simulink model "ve_model2"  (R2019a)
settings: Solver=FixedStepAuto  StartTime=0.0  StopTime=SimulationTime  FixedStep=IntegrationStep  RelTol=1e-3
model workspace (MAT data in the model file):
  IntegrationStep = 0.1
  SimulationTime = 0.1
  X0 = 0
  X_0 = 0
  Y0 = 0
  Y_0 = 0
  ang = 0.19739555985
  m = 1000
  vel = 3.14159265359
  xinitial = 1
libraries: autolibshared x1
settings Model: Creator=Vikas  LastModifiedBy=Vikas
settings DataIOCC: InitialState=xoutnew  LoadInitialState=on  SaveFinalState=on  SaveOperatingPoint=on  SaveState=on  StateSaveName=xoutnew  OutputSaveName=youtNew  ReturnWorkspaceOutputsName=SDOSimTest_Log
settings DebuggingCC: ArithmeticOperatorsInVariantConditions=warning

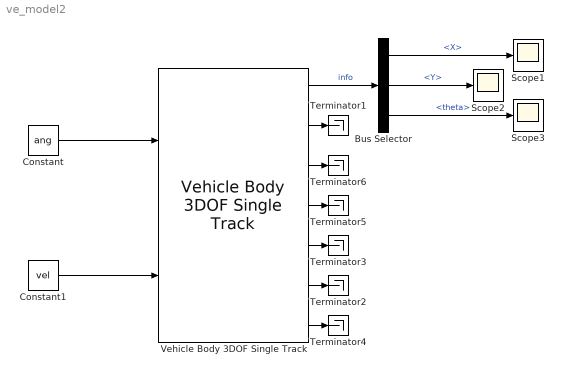
== system ve_model2 ==
  Bus Selector : BusSelector  OutputSignals=InertFrm.Cg.Disp.X,InertFrm.Cg.Disp.Y,InertFrm.Cg.Ang.theta
  Constant : Constant  Value=ang
  Constant1 : Constant  Value=vel
  Scope1 : Scope
  Scope2 : Scope
  Scope3 : Scope
  Terminator{1..6} (6 alike) : Terminator
  Vehicle Body 3DOF Single Track : autolibshared/Vehicle Body 3DOF Single Track  trackMode=Single (bicycle)  inputMode=External longitudinal velocity  frontSteerMode=on  rearSteerMode=off  windMode=off  muMode=off  extFMode=off  extMMode=off  extXo=off  extpsio=off  extxdoto=off  extro=off  extYo=off  extTamb=off  extydoto=off  aMode=2  NF=2  NR=2  m=m  a=1.4  b=1.6  h=0.35  X_o=X_0  xdot_o=0  CalphaMode=off  sigmaMode=on  d=0  w=[1.4,1.4]  Cy_f=12e3  Cy_r=11e3  sigma_f=.1  sigma_r=.1  alpha_f_brk=[-.1 .1]  Cy_f_data=[-9e3 9e3]  alpha_r_brk=[-.1 .1]  Cy_r_data=[-9e3 9e3]  Y_o=Y_0  ydot_o=0  Izz=4000  psi_o=0  r_o=0  Af=2  Cd=.3  Cl=.1  Cpm=.1  beta_w=[0:0.01:0.3]  Cs=[0:0.03:0.9]  Cym=[0:0.01:0.3]  Pabs=101325  Tair=273  g=9.81  mu=1  xdot_tol=.01  Fznom=5000  Fxtire_sat=7e4  Fytire_sat=7e4  longOff=0  latOff=0  vertOff=0  wrapAng=off
      settings: SourceProductName=Powertrain Blockset  SourceProductBaseCode=PW
  wires:
  Constant1/1 -> Vehicle Body 3DOF Single Track/2
  Vehicle Body 3DOF Single Track/6 -> Terminator2/1
  Vehicle Body 3DOF Single Track/7 -> Terminator4/1
  Vehicle Body 3DOF Single Track/5 -> Terminator3/1
  Vehicle Body 3DOF Single Track/4 -> Terminator5/1
  Vehicle Body 3DOF Single Track/3 -> Terminator6/1
  Vehicle Body 3DOF Single Track/1 -> Bus Selector/1  "info"
  Bus Selector/1 -> Scope1/1  "<X>"
  Bus Selector/2 -> Scope2/1  "<Y>"
  Bus Selector/3 -> Scope3/1  "<theta>"
  Vehicle Body 3DOF Single Track/2 -> Terminator1/1
  Constant/1 -> Vehicle Body 3DOF Single Track/1
